simulink model "Reference_Model_Subsystem1"  (R2020b)
settings: Solver=FixedStepAuto  StartTime=0.0  StopTime=10.0  FixedStep=0.2  RelTol=1e-3
settings Model: Creator=Sourav Kumar  LastModifiedBy=Sourav Kumar
settings DataIOCC: SaveOutput=off  SaveTime=off

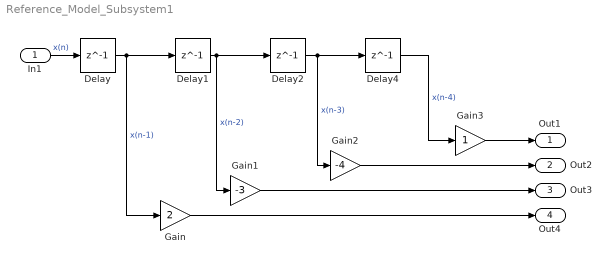
== system Reference_Model_Subsystem1 ==
  In1 : Inport  OutDataTypeStr=double  PortDimensions=1  SampleTime=[0,1]
  Delay{,1..2,4} (4 alike) : Delay  DelayLength=1
  Gain : Gain  Gain=2
  Gain1 : Gain  Gain=-3
  Gain2 : Gain  Gain=-4
  Gain3 : Gain
  Out1 : Outport  OutDataTypeStr=double  PortDimensions=1  SampleTime=[0.20000000000000001,0]
  Out2 : Outport  Port=2  OutDataTypeStr=double  PortDimensions=1  SampleTime=[0.20000000000000001,0]
  Out3 : Outport  Port=3  OutDataTypeStr=double  PortDimensions=1  SampleTime=[0.20000000000000001,0]
  Out4 : Outport  Port=4  OutDataTypeStr=double  PortDimensions=1  SampleTime=[0.20000000000000001,0]
  wires:
  Delay/1 -> Gain/1, Delay1/1  "x(n-1)"
  Delay4/1 -> Gain3/1  "x(n-4)"
  Gain1/1 -> Out3/1
  Gain/1 -> Out4/1
  Delay2/1 -> Delay4/1, Gain2/1  "x(n-3)"
  Delay1/1 -> Delay2/1, Gain1/1  "x(n-2)"
  In1/1 -> Delay/1  "x(n)"
  Gain2/1 -> Out2/1
  Gain3/1 -> Out1/1
